simulink model "winter_simulink"  (R2022a)
settings: Solver=FixedStepAuto  StartTime=0.0  StopTime=300  FixedStep=sample_time/10  RelTol=1e-3
values from neighbouring files (symbols this model uses):
  I_eq = rotor.I/gearbox.ratio^2 + generator.I    [main.m]
  sample_time = wind_speed(2,1) - wind_speed(1, 1)    [main.m]
undefined symbols (not defined in the file or in its folder): generator, omega_r, rotor
settings Model: Creator=Niccolò  LastModifiedBy=Niccolò

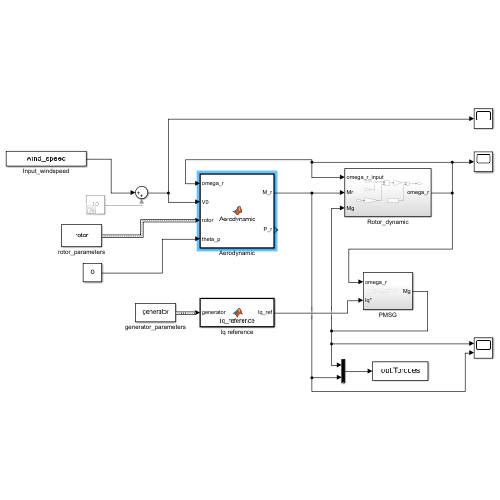
[thumbnail: Simulink's stored preview of the top-level diagram]
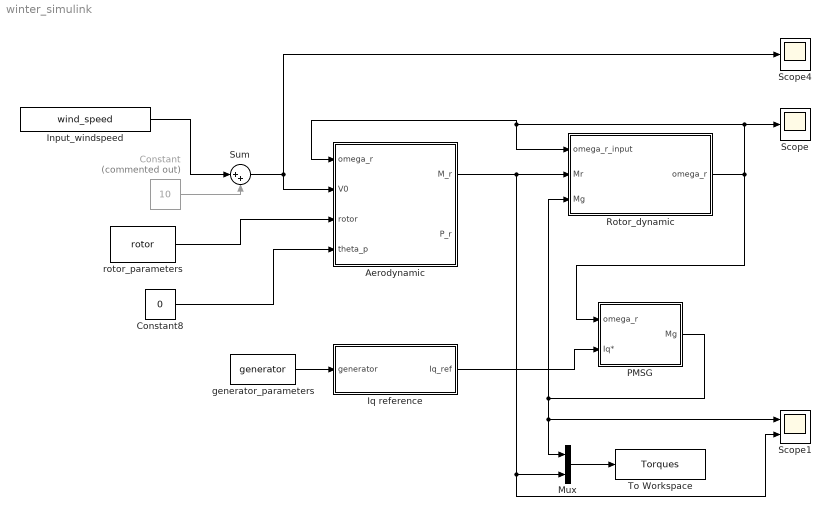
== system winter_simulink ==
  Aerodynamic : MATLAB Function  TreatAsAtomicUnit=on
  Constant : Constant  Commented=on  Value=10
  Constant8 : Constant  Value=0
  Input_windspeed : FromWorkspace  VariableName=wind_speed  SampleTime=sample_time
  Iq reference : MATLAB Function  TreatAsAtomicUnit=on
  Mux : Mux  Inputs=2
  PMSG : Subsystem
  Rotor_dynamic : Subsystem
  Scope : Scope
  Scope1 : Scope  NumInputPorts=2
  Scope4 : Scope
  Sum : Sum  Inputs=|++
  To Workspace : ToWorkspace  VariableName=Torques  SampleTime=-1
  generator_parameters : Constant  Value=generator  OutDataTypeStr=Bus: generator_bus
  rotor_parameters : Constant  Value=rotor  OutDataTypeStr=Bus: rotor_bus
  wires:
  Aerodynamic/1(M_r) -> Rotor_dynamic/2(Mr), Scope1/2, Mux/2
  PMSG/1(Mg) -> Scope1/1, Mux/1, Rotor_dynamic/3(Mg)
  Input_windspeed/1 -> Sum/1
  Constant/1 -> Sum/2
  Sum/1 -> Scope4/1, Aerodynamic/2(V0)
  Rotor_dynamic/1(omega_r) -> PMSG/1(omega_r), Aerodynamic/1(omega_r), Rotor_dynamic/1(omega_r_input), Scope/1
  Mux/1 -> To Workspace/1
  Constant8/1 -> Aerodynamic/4(theta_p)
  rotor_parameters/1 -> Aerodynamic/3(rotor)
  generator_parameters/1 -> Iq reference/1(generator)
  Iq reference/1(Iq_ref) -> PMSG/2(Iq*)

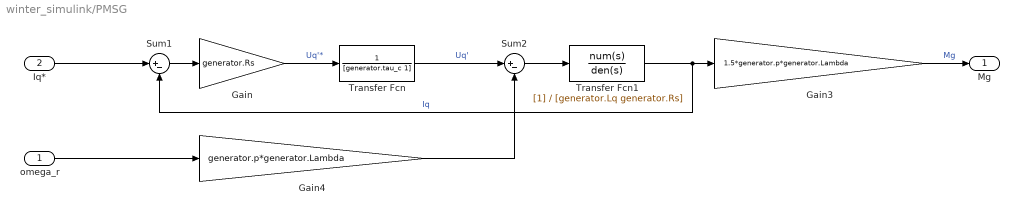
== system winter_simulink/PMSG ==
  omega_r : Inport
  Iq* : Inport  Port=2
  Gain : Gain  Gain=generator.Rs
  Gain3 : Gain  Gain=1.5*generator.p*generator.Lambda
  Gain4 : Gain  Gain=generator.p*generator.Lambda
  Sum1 : Sum  Inputs=|+-
  Sum2 : Sum  Inputs=|+-
  Transfer Fcn : TransferFcn  Denominator=[generator.tau_c 1]
  Transfer Fcn1 : TransferFcn  Denominator=[generator.Lq generator.Rs]
  Mg : Outport
  wires:
  Sum2/1 -> Transfer Fcn1/1
  omega_r/1 -> Gain4/1
  Transfer Fcn1/1 -> Sum1/2, Gain3/1  "Iq"
  Sum1/1 -> Gain/1
  Transfer Fcn/1 -> Sum2/1  "Uq'"
  Gain/1 -> Transfer Fcn/1  "Uq'*"
  Gain4/1 -> Sum2/2
  Gain3/1 -> Mg/1  "Mg"
  Iq*/1 -> Sum1/1

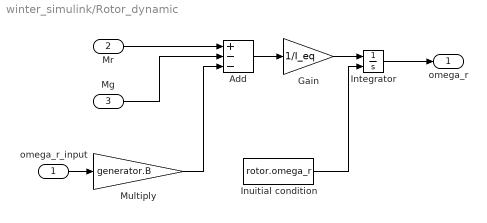
== system winter_simulink/Rotor_dynamic ==
  omega_r_input : Inport
  Mr : Inport  Port=2
  Mg : Inport  Port=3
  Add : Sum  Inputs=+--
  Gain : Gain  Gain=1/I_eq
  Integrator : Integrator  InitialConditionSource=external  InitialCondition=omega_r
  Inuitial condition : Constant  Value=rotor.omega_r
  Multiply : Gain  Gain=generator.B
  omega_r : Outport
  wires:
  Add/1 -> Gain/1
  Gain/1 -> Integrator/1
  Mr/1 -> Add/1
  Integrator/1 -> omega_r/1
  Mg/1 -> Add/2
  Inuitial condition/1 -> Integrator/2
  omega_r_input/1 -> Multiply/1
  Multiply/1 -> Add/3

== matlab function winter_simulink/Iq reference ==
  data: generator input; Iq_ref output
function Iq_ref = Iq_reference(generator)

Lambda = generator.Lambda;
p = generator.p;
Tg = 1000;% interp1( );
Iq_ref = Tg/(1.5*p*Lambda);

== matlab function winter_simulink/Aerodynamic ==
  data: omega_r input; V0 input; M_r output; P_r output; rho parameter; rotor input; theta_p input
function [M_r, P_r] = Aerodynamic(omega_r, V0, rho, rotor, theta_p) 

R = rotor.R;                  % rotor radius [m]

% retrive the cP from the look-up table
lambda = omega_r*R/V0;                                                
cP = interp2(lambda_vector, pitch_vector, cP_store, lambda, theta_p);

P_r = 0.5*rho*V0^3*pi*R^2*cP; % rotor power [W]
M_r = P_r/omega_r;                                    % rotor torque [Nm]
